simulink model "assign1"  (R2020b)
settings: Solver=VariableStepAuto  StartTime=0.0  StopTime=40  RelTol=1e-3
values from neighbouring files (symbols this model uses):
  A = [4,1,-2;1,0,2;1,-1,3]    [test.m]    (also in test2.m = [1 0 0 0;2 -3 0 0;1 0 -2 0;4 -1 -2 -4]; test3.m = [-1 0 0 0;2 -3 0 0;0 0 2 0;4 -1 2 -4])
  B = [3,1;2,7;5,3]    [test.m]    (also in test2.m = [0;0;1;2]; test3.m = [0 0 1 2]')
  C = [1,2,0;0,1,1]    [test.m]    (also in test2.m = [3 0 1 0]; test3.m = [3 0 1 0])
  D = [0,0;0,0]    [test.m]    (also in test3.m = [0])
settings Model: Creator=10911  LastModifiedBy=10911

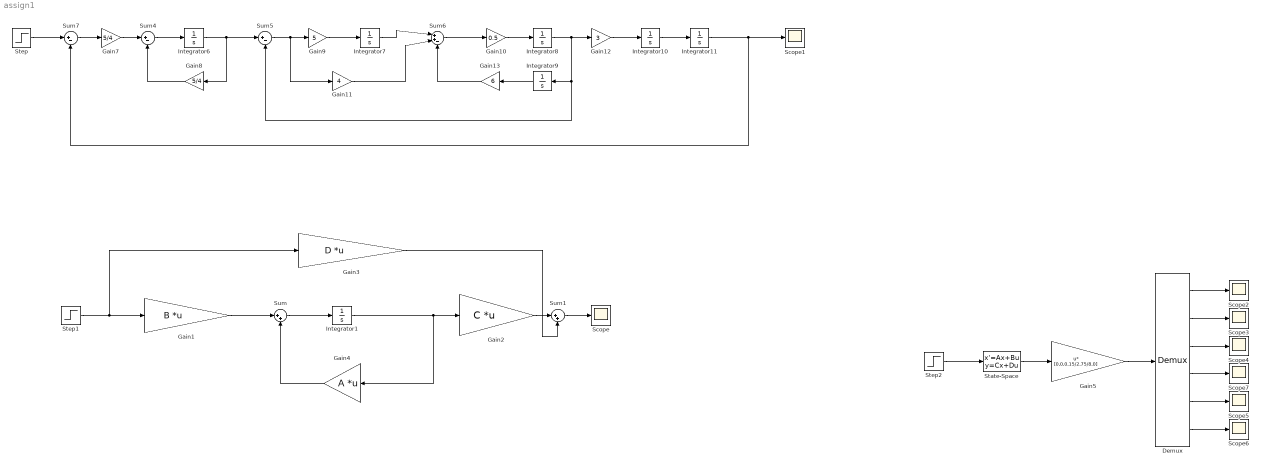
== system assign1 ==
  Demux : Demux  Outputs=6
  Gain1 : Gain  Gain=B  Multiplication=Matrix(K*u)
  Gain10 : Gain  Gain=0.5
  Gain11 : Gain  Gain=4
  Gain12 : Gain  Gain=3
  Gain13 : Gain  Gain=6
  Gain2 : Gain  Gain=C  Multiplication=Matrix(K*u)
  Gain3 : Gain  Gain=D  Multiplication=Matrix(K*u)
  Gain4 : Gain  Gain=A  Multiplication=Matrix(K*u)
  Gain5 : Gain  Gain=[0,0,0,15/2,75/8,0]  Multiplication=Matrix(u*K)
  Gain7 : Gain  Gain=5/4
  Gain8 : Gain  Gain=5/4
  Gain9 : Gain  Gain=5
  Integrator{1,6..11} (7 alike) : Integrator
  Scope{,1..7} (8 alike) : Scope
  State-Space : StateSpace  A=[-13/4,-8,-55/8,-15/2,-75/8,0;1,0,0,0,0,0;0,1,0,0,0,0;0,0,1,0,0,0;0,0,0,1,0,0;0,0,0,0,1,0]  B=[1;0;0;0;0;0]  C=[0,0,0,15/2,75/8,0]  D=0  InitialCondition=0
  Step : Step  SampleTime=0
  Step1 : Step  SampleTime=0
  Step2 : Step  SampleTime=0
  Sum : Sum  Inputs=|++
  Sum1 : Sum  Inputs=|++
  Sum4 : Sum  Inputs=|+-
  Sum5 : Sum  Inputs=|+-
  Sum6 : Sum  Inputs=|++-
  Sum7 : Sum  Inputs=|+-
  wires:
  Step/1 -> Sum7/1
  Sum7/1 -> Gain7/1
  Gain13/1 -> Sum6/3
  Gain9/1 -> Integrator7/1
  Integrator9/1 -> Gain13/1
  Gain11/1 -> Sum6/2
  Sum5/1 -> Gain11/1, Gain9/1
  Sum6/1 -> Gain10/1
  Gain10/1 -> Integrator8/1
  Integrator10/1 -> Integrator11/1
  Integrator6/1 -> Gain8/1, Sum5/1
  Gain8/1 -> Sum4/2
  Integrator8/1 -> Sum5/2, Integrator9/1, Gain12/1
  Sum4/1 -> Integrator6/1
  Gain7/1 -> Sum4/1
  Gain12/1 -> Integrator10/1
  Integrator7/1 -> Sum6/1
  Integrator11/1 -> Sum7/2, Scope1/1
  Step1/1 -> Gain3/1, Gain1/1
  Gain1/1 -> Sum/1
  Sum/1 -> Integrator1/1
  Integrator1/1 -> Gain2/1, Gain4/1
  Gain2/1 -> Sum1/1
  Sum1/1 -> Scope/1
  Gain3/1 -> Sum1/2
  Gain4/1 -> Sum/2
  Step2/1 -> State-Space/1
  Gain5/1 -> Demux/1
  State-Space/1 -> Gain5/1
  Demux/1 -> Scope2/1
  Demux/2 -> Scope3/1
  Demux/3 -> Scope4/1
  Demux/4 -> Scope7/1
  Demux/5 -> Scope5/1
  Demux/6 -> Scope6/1
